simulink model "add_uss_mdl"  (R2013a)
settings: Solver=ode45  StartTime=0.0  StopTime=10.0  RelTol=1e-3
undefined symbols (not defined in the file or in its folder): add_usys_d
settings Model: Creator=Kostas  LastModifiedBy=Kostas

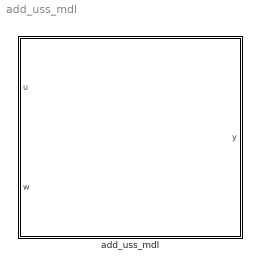
== system add_uss_mdl ==
  add_uss_mdl : Subsystem

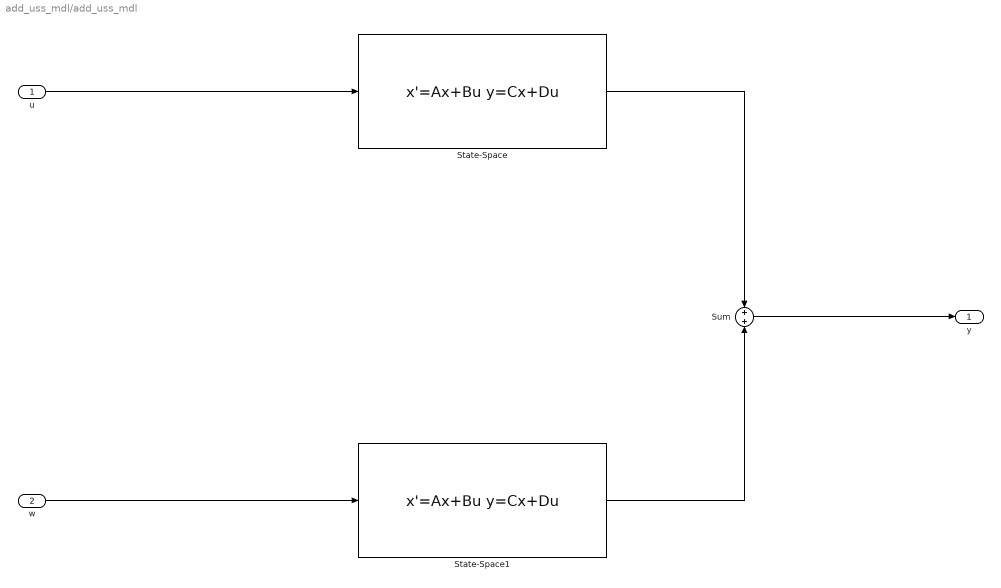
== system add_uss_mdl/add_uss_mdl ==
  u : Inport
  w : Inport  Port=2
  State-Space : StateSpace  A=add_usys_d.continuous.matrices.A  B=add_usys_d.continuous.matrices.B  C=add_usys_d.continuous.matrices.C  D=add_usys_d.continuous.matrices.D
  State-Space1 : StateSpace  A=add_usys_d.continuous.matrices.A  B=add_usys_d.continuous.matrices.E  C=add_usys_d.continuous.matrices.C  D=add_usys_d.continuous.matrices.D
  Sum : Sum  Inputs=+|+
  y : Outport
  wires:
  u/1 -> State-Space/1
  w/1 -> State-Space1/1
  State-Space/1 -> Sum/1
  State-Space1/1 -> Sum/2
  Sum/1 -> y/1
